simulink subsystem "DCEquivalentFaulhaber_2214_024_BXTH"  (R2024a)
settings: Solver=VariableStepAuto  StartTime=0.0  StopTime=10.0  RelTol=1e-3
libraries: ee_lib x1, fl_lib x1
settings Model: DataDictionary=neck_mk3.sldd  EnableAccessToBaseWorkspace=off  Creator=upattacini  LastModifiedBy=upattacini
settings RTWCC: GPUComputeCapability=3.5

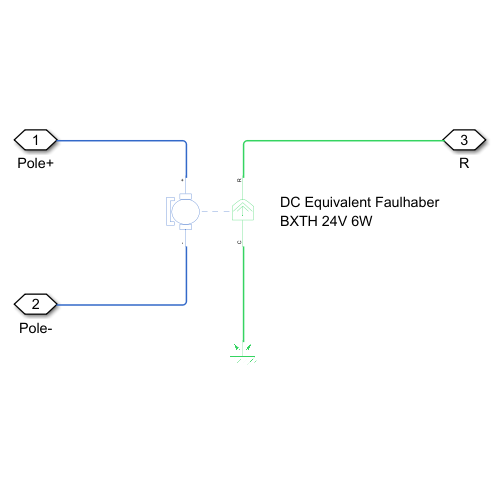
[thumbnail: Simulink's stored preview of the top-level diagram]
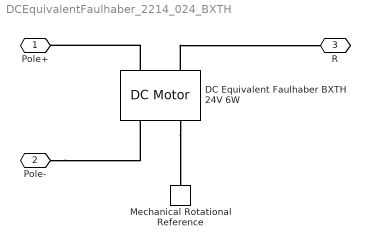
== system DCEquivalentFaulhaber_2214_024_BXTH ==
  DC Equivalent Faulhaber BXTH 24V 6W : ee_lib/Electromechanical/Brushed Motors/DC Motor  field_option=ee.enum.field_option.pm  Rf=100 Ohm  Lf=1 H  Laf=0.15 H  If0=0 A  parameterization=ee.enum.dcparam_option.circuit_param  Ra=25.9 / 2 Ohm  La=3150 uH  emf_or_torque=ee.enum.emf_or_torque.ki  Kv=0.072e-3 V/rpm  Ki=32.2 * sqrt(3/2) m*mN/A  T_stall=0.24e-3 N*m  w_max=19100 rpm  w_rated=15000 rpm  P_rated=0.08 W  V_rated=48 V  lam_param=ee.enum.lam_param.current  i_noload=0.016 A  V_i_noload=24 V  J=3.3 cm^2*g  lam=0.0010099 N*m*s/rad  speed0=0 rpm  enable_fault_armature=simscape.enum.onoff.off  rev_faulted=1 / 3  G_faulted_armature=1e-5 S  fault_trigger_armature=ee.enum.faults.faultTrigger.temporal  t_fault_armature=1 s  max_permissible_current_armature=inf A  t_fail_on_current_armature=1 s  enable_fault_field=simscape.enum.onoff.off  G_faulted_field=1e-5 S  fault_trigger_field=ee.enum.faults.faultTrigger.temporal  t_fault_field=1 s  max_permissible_current_field=inf A  t_fail_on_current_field=1 s  fault_action=simscape.enum.assert.action.none  alpha=3.93e-3 1/K  Tmeas=25 degC  thermal_mass=100 J/K  initial_temperature=25 degC
  Mechanical Rotational Reference : fl_lib/Mechanical/Rotational Elements/Mechanical Rotational Reference
  Pole+ : PMIOPort  Side=Left
  Pole- : PMIOPort  Port=2  Side=Left
  R : PMIOPort  Port=3  Side=Right
  connections:
  DC Equivalent Faulhaber BXTH 24V 6W/RConn2 -- Mechanical Rotational Reference/LConn1
  DC Equivalent Faulhaber BXTH 24V 6W/LConn1 -- Pole+/RConn1
  DC Equivalent Faulhaber BXTH 24V 6W/LConn2 -- R/RConn1
  Pole-/RConn1 -- DC Equivalent Faulhaber BXTH 24V 6W/RConn1
